simulink library "pixhawk_slib_adv"  (R2017b)
settings: Solver=ode45  StartTime=0.0  StopTime=10.0  RelTol=1e-3
undefined symbols (not defined in the file or in its folder): Earth, earthRadius, ModelInit_AngEuler, ModelInit_PosE, ModelInit_RateB, ModelInit_RPM, ModelInit_VelB, ModelParam_envAltitude, ModelParam_GPSLatLong, ModelParam_motorCr, ModelParam_motorJm, ModelParam_motorT, ModelParam_motorWb, ModelParam_noisePowerIMU, ModelParam_rotorCm, ModelParam_rotorCt, ModelParam_uavCCm, ModelParam_uavCd, ModelParam_uavDearo, ModelParam_uavJ, ModelParam_uavMass, ModelParam_uavR, ModelParam_uavType, Receive, Send, WGS84
libraries: etargetslib x11, dspnetwork x9, simulink x8, sharedtransform x5, aerolibtransform2 x4, aerolibutil x4, pixhawk_slib_adv x3, aerolibfltsims x3, shared6dof x1, aerolibobsolete x1, aerolibasang x1, aerolibatmos2 x1
(part 1 of 3)
settings Model: Creator=skuznick  LastModifiedBy=uavcs
settings DataIOCC: LimitDataPoints=on  SaveFormat=Array
settings OptimizationCC: BlockReduction=off  BooleanDataType=off  LifeSpan=inf
settings DebuggingCC: SaveWithParameterizedLinksMsg=none  UnderspecifiedInitializationDetection=Classic  MergeDetectMultiDrivingBlocksExec=none  SignalResolutionControl=TryResolveAllWithWarning  AllowSymbolicDim=off  SFUnexpectedBacktrackingDiag=warning  SFNoUnconditionalDefaultTransitionDiag=warning  SFExecutionAtInitializationDiag=none
settings HardwareCC: ProdBitPerPointer=32  ProdBitPerSizeT=32  ProdBitPerPtrDiffT=32  ProdLargestAtomicFloat=None  ProdIntDivRoundTo=Undefined  ProdEndianess=Unspecified  ProdWordSize=32  ProdHWDeviceType=32-bit Generic  TargetUnknown=on
settings ModelReferenceCC: PropagateSignalLabelsOutOfModel=off
settings CodeAppCC: StateflowObjectComments=on
settings GRTTargetCC: TargetLangStandard=C89/C90 (ANSI)
settings ConfigComp: CovMetricSettings=dw  CovSaveCumulativeToWorkspaceVar=on  CovSaveSingleToWorkspaceVar=on  CovExternalEMLEnable=off  CovSFcnEnable=off

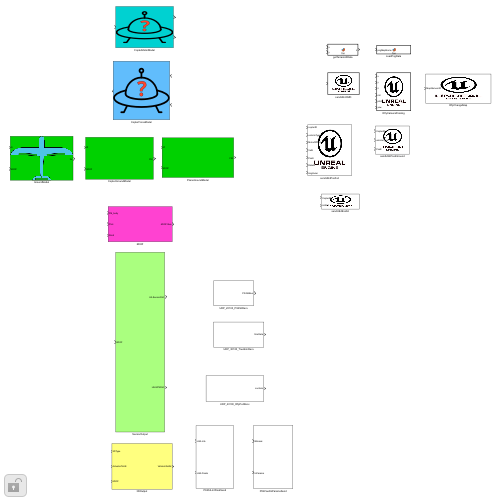
[thumbnail: Simulink's stored preview of the top-level diagram]
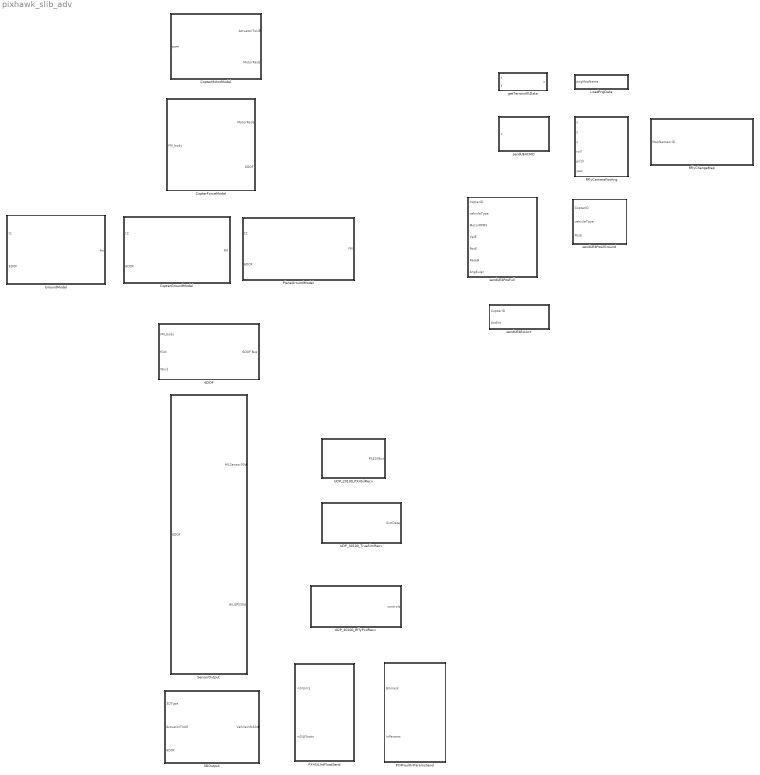
== system pixhawk_slib_adv ==
  3DOutput : Subsystem  mask(3DOutput API){}
      mask help:
      | 该模块输入为：
      | 1）UAVType：三维显示ID，来自***_init.m中的ModelParam_uavType，由三维模型文件中的XML文件决定，例如：常规四旋翼的UAVType为3，小型固定翼的UAVType为100。
      | 2）ActuatorToUE：来自电机模型，决定了在三维引擎中无人载具系统电机/舵机的转动情况。
      | 3）6DOF：来自6DOF模型的6DOF Bus输入，接收无人载具系统的位置、速度、姿态和加速度等信息。
      | 输出为VehileInfo60d：在三维显示模块中，会通过该接口将数据发送至三维引擎，实现可视化处理。
      mask Help: eval('sharedhelp(''3doutput'')');
      mask DialogControl Control3 Prompt: 模块详解
      mask DialogControl Control3 Callback: !start ../html/md_ctrl_2md_23DOutput.html
      mask DialogControl Control2 Prompt: (Add text here)
  6DOF : Subsystem  mask(6DOF API){Init_PosE=ModelInit_PosE, Init_VelB=ModelInit_VelB, Init_AngEuler=ModelInit_AngEuler, Init_RateB=ModelInit_RateB, Param_uavMass=ModelParam_uavMass, Param_uavJ=ModelParam_uavJ, Param_GPSLatLong=ModelParam_GPSLatLong, Param_envAltitude=ModelParam_envAltitude}
      mask prompts: Init_PosE "Initial position NED:"; Init_VelB "Initial velocity FRD:"; Init_AngEuler "Initial Euler Ang:"; Init_RateB "Initial Ang Rate:"; Param_uavMass "Vehilce Mass:"; Param_uavJ "Vehicle Inertial Matrix:"; Param_GPSLatLong "Gps Initial Lat and Lon:"; Param_envAltitude "Gps Init Alt:"
      mask help:
      | 该模块中包括了环境模型和基于四元数的刚体六自由度模型。环境模型对重力和大气压强对无人系统飞行产生的影响进行了模拟；刚体六自由度模型用于描述无人载具运动时的姿态和位置变化
      | 以旋翼无人机为例，六自由度模块基于刚体动力学原理，将无人机视为一个刚体，并考虑了无人机在三个坐标轴上的旋转运动（俯仰、横滚和偏航）以及机体与地球坐标系上的平移运动（前后、左右和上下）。
      | 该模块通过对这些自由度进行数学建模，可以推导出无人机在空中运动时的动力学方程，从而可以进行控制系统设计、路径规划和飞行模拟等应用。此外，还可以根据实际需求对模型进行扩展，考虑更多的因素，如飞行器的非线性特性、气动力和惯性矩等。
      | 该模型的输入为机体所受的力和力矩，输出为机体坐标系下的速度与加速度，地球坐标系下的速度，位置，欧拉角，方向余弦矩阵（旋转矩阵），角速度与角加速度。
      mask Help: eval('sharedhelp(''6dof'')');
      mask DialogControl Control2 Prompt: 模块详解
      mask DialogControl Control2 Callback: !start ../html/md_ctrl_2md_26DOF.html
  CopterForceModel : Subsystem  mask(CopterForceModel){AirframeChoice=default, Param_uavType=ModelParam_uavType, Param_uavR=ModelParam_uavR, Param_motorJm=ModelParam_motorJm, Param_rotorCm=ModelParam_rotorCm, Param_rotorCt=ModelParam_rotorCt, Param_uavCd=ModelParam_uavCd, Param_uavCCm=ModelParam_uavCCm, Param_uavDearo=ModelParam_uavDearo}
      mask prompts: Param_uavType "Uav type id:"; Param_uavR "Airframe size:"; Param_motorJm "Propeller Jm:"; Param_rotorCm "Propeller Cm:"; Param_rotorCt "Propeller Ct:"; Param_uavCd "Uav Cd:"; Param_uavCCm "Uav Cm:"; Param_uavDearo "Uav d_aero:"
      mask help: 力和力矩子系统主要用于综合执行器状态、飞行环境状态和机体运动状态，来计算出机身子系统受到的合力和力矩。为了方便六自由度机体运动模型的使用，合力和力矩通常需要统一映射（坐标转换）到机体坐标系中。
      mask init:
      | choice = get_param(gcb, 'AirframeChoice');
      | switch choice
      |     case 'default'
      |         set_param(gcb, 'Param_uavType', 'ModelParam_uavType');
      |         set_param(gcb, 'Param_uavR', 'ModelParam_uavR');
      |         set_param(gcb, 'Param_motorJm', 'ModelParam_motorJm');
      |         set_param(gcb, 'Param_rotorCm', 'ModelParam_rotorCm');
      |         set_param(gcb, 'Param_rotorCt', 'ModelParam_rotorCt');
      |         set_param(gcb, 'Param_uavCd', 'ModelParam_uavCd');
      |         set_param(gcb, 'Param_uavDearo', 'ModelParam_uavDearo');
      |         set_param(gcb, 'Param_uavCCm', 'ModelParam_uavCCm');
      |     case 'Tricopter Y+'
      |         Param_uavType=int16(1)
      |         Param_uavR=0.225
      |         Param_motorJm=2.13e-4
      |         Param_rotorCm=1.789e-7
      |         Param_rotorCt=1.051e-5
      |         Param_uavCd=0.227
      |         Param_uavDearo=0.12
      |         Param_uavCCm=[0.0035; 0.0039; 0.0034]
      |         set_param(gcb, 'Param_uavCCm', mat2str(Param_uavCCm,'class'));
      |         set_param(gcb, 'Param_uavType', num2str(Param_uavType));
      |         set_param(gcb, 'Param_uavR', num2str(Param_uavR));
      |         set_param(gcb, 'Param_motorJm', num2str(Param_motorJm));
      |         set_param(gcb, 'Param_rotorCm', num2str(Param_rotorCm));
      |         set_param(gcb, 'Param_rotorCt', num2str(Param_rotorCt));
      |         set_param(gcb, 'Param_uavCd', num2str(Param_uavCd));
      |         set_param(gcb, 'Param_uavDearo', num2str(Param_uavDearo));
      |     case 'Tricopter Y-'
      |         Param_uavType=int16(2)
      |         Param_uavR=0.225
      |         Param_motorJm=2.13e-4
      |         Param_rotorCm=1.789e-7
      |         Param_rotorCt=1.051e-5
      |         Param_uavCd=0.227
      |         Param_uavDearo=0.12
      |         Param_uavCCm=[0.0035; 0.0039; 0.0034]
      |         set_param(gcb, 'Param_uavCCm', mat2str(Param_uavCCm,'class'));
      |         set_param(gcb, 'Param_uavType', num2str(Param_uavType));
      |         set_param(gcb, 'Param_uavR', num2str(Param_uavR));
      |         set_param(gcb, 'Param_motorJm', num2str(Param_motorJm));
      |         set_param(gcb, 'Param_rotorCm', num2str(Param_rotorCm));
      |         set_param(gcb, 'Param_rotorCt', num2str(Param_rotorCt));
      |         set_param(gcb, 'Param_uavCd', num2str(Param_uavCd));
      |         set_param(gcb, 'Param_uavDearo', num2str(Param_uavDearo));
      |     case 'Quadrotor X'
      |         Param_uavType=int16(3)
      |         Param_uavR=0.225
      |         Param_motorJm=0.0001287
      |         Param_rotorCm=2.783e-07
      |         Param_rotorCt=1.681e-05
      |         Param_uavCd=0.055
      |         Param_uavDearo=0.12
      |         Param_uavCCm=[0.0035; 0.0039; 0.0034]
      |         set_param(gcb, 'Param_uavCCm', mat2str(Param_uavCCm,'class'));
      |         set_param(gcb, 'Param_uavType', num2str(Param_uavType));
      |         set_param(gcb, 'Param_uavR', num2str(Param_uavR));
      |         set_param(gcb, 'Param_motorJm', num2str(Param_motorJm));
      |         set_param(gcb, 'Param_rotorCm', num2str(Param_rotorCm));
      |         set_param(gcb, 'Param_rotorCt', num2str(Param_rotorCt));
      |         set_param(gcb, 'Param_uavCd', num2str(Param_uavCd));
      |         set_param(gcb, 'Param_uavDearo', num2str(Param_uavDearo));
      |     case 'Quadrotor +'
      |         Param_uavType=int16(4)
      |         Param_uavR=0.225
      |         Param_motorJm=0.0001287
      |         Param_rotorCm=2.783e-07
      |         Param_rotorCt=1.681e-05
      |         Param_uavCd=0.055
      |         Param_uavDearo=0.12
      |         Param_uavCCm=[0.0035; 0.0039; 0.0034]
      |         set_param(gcb, 'Param_uavCCm', mat2str(Param_uavCCm,'class'));
      |         set_param(gcb, 'Param_uavType', num2str(Param_uavType));
      |         set_param(gcb, 'Param_uavR', num2str(Param_uavR));
      |         set_param(gcb, 'Param_motorJm', num2str(Param_motorJm));
      |         set_param(gcb, 'Param_rotorCm', num2str(Param_rotorCm));
      |         set_param(gcb, 'Param_rotorCt', num2str(Param_rotorCt));
      |         set_param(gcb, 'Param_uavCd', num2str(Param_uavCd));
      |         set_param(gcb, 'Param_uavDearo', num2str(Param_uavDearo));
      |     case 'Hexarotor x'
      |         Param_uavType=int16(5)
      |         Param_uavR=0.275
      |         Param_motorJm=2.13e-4
      |         Param_rotorCm=1.789e-7 
      |         Param_rotorCt=1.051e-5 
      |         Param_uavCd=0.339
      |         Param_uavDearo=0.12
      |         Param_uavCCm=[0.0035; 0.0039; 0.0034]
      |         set_param(gcb, 'Param_uavCCm', mat2str(Param_uavCCm,'class'));
      |         set_param(gcb, 'Param_uavType', num2str(Param_uavType));
      |         set_param(gcb, 'Param_uavR', num2str(Param_uavR));
      |         set_param(gcb, 'Param_motorJm', num2str(Param_motorJm));
      |         set_param(gcb, 'Param_rotorCm', num2str(Param_rotorCm));
      |         set_param(gcb, 'Param_rotorCt', num2str(Param_rotorCt));
      |         set_param(gcb, 'Param_uavCd', num2str(Param_uavCd));
      |         set_param(gcb, 'Param_uavDearo', num2str(Param_uavDearo));
      |     case 'Hexarotor +'
      |         Param_uavType=int16(6)
      |         Param_uavR=0.275
      |         Param_motorJm=2.13e-4
      |         Param_rotorCm=1.789e-7 
      |         Param_rotorCt=1.051e-5 
      |         Param_uavCd=0.339
      |         Param_uavDearo=0.12
      |         Param_uavCCm=[0.0035; 0.0039; 0.0034]
      |         set_param(gcb, 'Param_uavCCm', mat2str(Param_uavCCm,'class'));
      |         set_param(gcb, 'Param_uavType', num2str(Param_uavType));
      |         set_param(gcb, 'Param_uavR', num2str(Param_uavR));
      |         set_param(gcb, 'Param_motorJm', num2str(Param_motorJm));
      |         set_param(gcb, 'Param_rotorCm', num2str(Param_rotorCm));
      |         set_param(gcb, 'Param_rotorCt', num2str(Param_rotorCt));
      |         set_param(gcb, 'Param_uavCd', num2str(Param_uavCd));
      |         set_param(gcb, 'Param_uavDearo', num2str(Param_uavDearo));
      |     case 'Hexarotor Coaxial'
      |         Param_uavType=int16(7)
      |         Param_uavR=0.225
      |         Param_motorJm=2.13e-4 
      |         Param_rotorCm=1.789e-7
      |         Param_rotorCt=1.051e-5
      |         Param_uavCd=0.228 
      |         Param_uavDearo=0.12
      |         Param_uavCCm=[0.0035; 0.0039; 0.0034]
      |         set_param(gcb, 'Param_uavCCm', mat2str(Param_uavCCm,'class'));
      |         set_param(gcb, 'Param_uavType', num2str(Param_uavType));
      |         set_param(gcb, 'Param_uavR', num2str(Param_uavR));
      |         set_param(gcb, 'Param_motorJm', num2str(Param_motorJm));
      |         set_param(gcb, 'Param_rotorCm', num2str(Param_rotorCm));
      |         set_param(gcb, 'Param_rotorCt', num2str(Param_rotorCt));
      |         set_param(gcb, 'Param_uavCd', num2str(Param_uavCd));
      |         set_param(gcb, 'Param_uavDearo', num2str(Param_uavDearo));
      |     case 'Octorotor x'
      |         Param_uavType=int16(8)
      |         Param_uavR=0.325
      |         Param_motorJm= 8.00e-5 
      |         Param_rotorCm= 1.417e-7
      |         Param_rotorCt=8.380e-6
      |         Param_uavCd=0.472
      |         Param_uavDearo=0.12
      |         Param_uavCCm=[0.0035; 0.0039; 0.0034]
      |         set_param(gcb, 'Param_uavCCm', mat2str(Param_uavCCm,'class'));
      |         set_param(gcb, 'Param_uavType', num2str(Param_uavType));
      |         set_param(gcb, 'Param_uavR', num2str(Param_uavR));
      |         set_param(gcb, 'Param_motorJm', num2str(Param_motorJm));
      |         set_param(gcb, 'Param_rotorCm', num2str(Param_rotorCm));
      |         set_param(gcb, 'Param_rotorCt', num2str(Param_rotorCt));
      |         set_param(gcb, 'Param_uavCd', num2str(Param_uavCd));
      |         set_param(gcb, 'Param_uavDearo', num2str(Param_uavDearo));
      |     case 'Octorotor +'
      |         Param_uavType=int16(9)
      |         Param_uavR=0.325
      |         Param_motorJm= 8.00e-5 
      |         Param_rotorCm= 1.417e-7
      |         Param_rotorCt=8.380e-6
      |         Param_uavCd=0.472
      |         Param_uavDearo=0.12
      |         Param_uavCCm=[0.0035; 0.0039; 0.0034]
      |         set_param(gcb, 'Param_uavCCm', mat2str(Param_uavCCm,'class'));
      |         set_param(gcb, 'Param_uavType', num2str(Param_uavType));
      |         set_param(gcb, 'Param_uavR', num2str(Param_uavR));
      |         set_param(gcb, 'Param_motorJm', num2str(Param_motorJm));
      |         set_param(gcb, 'Param_rotorCm', num2str(Param_rotorCm));
      |         set_param(gcb, 'Param_rotorCt', num2str(Param_rotorCt));
      |         set_param(gcb, 'Param_uavCd', num2str(Param_uavCd));
      |         set_param(gcb, 'Param_uavDearo', num2str(Param_uavDearo));
      |     case 'Octorotor Coaxial'
      |         Param_uavType=int16(10)
      |         Param_uavR=0.275
      |         Param_motorJm=2.13e-4 
      |         Param_rotorCm=1.789e-7 
      |         Param_rotorCt=1.051e-5 
      |         Param_uavCd=0.338
      |         Param_uavDearo=0.12
      |         Param_uavCCm=[0.0035; 0.0039; 0.0034]
      |         set_param(gcb, 'Param_uavCCm', mat2str(Param_uavCCm,'class'));
      |         set_param(gcb, 'Param_uavType', num2str(Param_uavType));
      |         set_param(gcb, 'Param_uavR', num2str(Param_uavR));
      |         set_param(gcb, 'Param_motorJm', num2str(Param_motorJm));
      |         set_param(gcb, 'Param_rotorCm', num2str(Param_rotorCm));
      |         set_param(gcb, 'Param_rotorCt', num2str(Param_rotorCt));
      |         set_param(gcb, 'Param_uavCd', num2str(Param_uavCd));
      |         set_param(gcb, 'Param_uavDearo', num2str(Param_uavDearo)); 
      |     otherwise
      |         error('Unknown AirframeChoice');
      | end
      | 
      | % 更新Param_uavType参数值
      | 
      | % 显示更新后的值在mask界面上（假设你有一个显示区域来展示此值）
      | disp(['Updated Param_uavType: ', num2str(Param_uavType)]);
      mask Help: eval('sharedhelp(''copterforce'')');
      mask TypeOptions AirframeChoice: default | Tricopter Y+ | Tricopter Y- | Quadrotor X | Quadrotor + | Hexarotor x | Hexarotor + | Hexarotor Coaxial | Octorotor x | Octorotor + | Octorotor Coaxial
      mask Callback AirframeChoice:
      | choice = get_param(gcb, 'AirframeChoice');
      | switch choice
      |     case 'default'
      |         set_param(gcb, 'Param_uavType', 'ModelParam_uavType');
      |         set_param(gcb, 'Param_uavR', 'ModelParam_uavR');
      |         set_param(gcb, 'Param_motorJm', 'ModelParam_motorJm');
      |         set_param(gcb, 'Param_rotorCm', 'ModelParam_rotorCm');
      |         set_param(gcb, 'Param_rotorCt', 'ModelParam_rotorCt');
      |         set_param(gcb, 'Param_uavCd', 'ModelParam_uavCd');
      |         set_param(gcb, 'Param_uavDearo', 'ModelParam_uavDearo');
      |         set_param(gcb, 'Param_uavCCm', 'ModelParam_uavCCm');
      |     case 'Tricopter Y+'
      |         Param_uavType=1
      |         Param_uavR=0.225
      |         Param_motorJm=2.13e-4
      |         Param_rotorCm=1.789e-7
      |         Param_rotorCt=1.051e-5
      |         Param_uavCd=0.227
      |         Param_uavDearo=0.12
      |         Param_uavCCm=[0.0035; 0.0039; 0.0034]
      |         set_param(gcb, 'Param_uavCCm', mat2str(Param_uavCCm,'class'));
      |         set_param(gcb, 'Param_uavType', num2str(Param_uavType));
      |         set_param(gcb, 'Param_uavR', num2str(Param_uavR));
      |         set_param(gcb, 'Param_motorJm', num2str(Param_motorJm));
      |         set_param(gcb, 'Param_rotorCm', num2str(Param_rotorCm));
      |         set_param(gcb, 'Param_rotorCt', num2str(Param_rotorCt));
      |         set_param(gcb, 'Param_uavCd', num2str(Param_uavCd));
      |         set_param(gcb, 'Param_uavDearo', num2str(Param_uavDearo));
      |     case 'Tricopter Y-'
      |         Param_uavType=2
      |         Param_uavR=0.225
      |         Param_motorJm=2.13e-4
      |         Param_rotorCm=1.789e-7
      |         Param_rotorCt=1.051e-5
      |         Param_uavCd=0.227
      |         Param_uavDearo=0.12
      |         Param_uavCCm=[0.0035; 0.0039; 0.0034]
      |         set_param(gcb, 'Param_uavCCm', mat2str(Param_uavCCm,'class'));
      |         set_param(gcb, 'Param_uavType', num2str(Param_uavType));
      |         set_param(gcb, 'Param_uavR', num2str(Param_uavR));
      |         set_param(gcb, 'Param_motorJm', num2str(Param_motorJm));
      |         set_param(gcb, 'Param_rotorCm', num2str(Param_rotorCm));
      |         set_param(gcb, 'Param_rotorCt', num2str(Param_rotorCt));
      |         set_param(gcb, 'Param_uavCd', num2str(Param_uavCd));
      |         set_param(gcb, 'Param_uavDearo', num2str(Param_uavDearo));
      |     case 'Quadrotor X'
      |         Param_uavType=3
      |         Param_uavR=0.225
      |         Param_motorJm=0.0001287
      |         Param_rotorCm=2.783e-07
      |         Param_rotorCt=1.681e-05
      |         Param_uavCd=0.055
      |         Param_uavDearo=0.12
      |         Param_uavCCm=[0.0035; 0.0039; 0.0034]
      |         set_param(gcb, 'Param_uavCCm', mat2str(Param_uavCCm,'class'));
      |         set_param(gcb, 'Param_uavType', num2str(Param_uavType));
      |         set_param(gcb, 'Param_uavR', num2str(Param_uavR));
      |         set_param(gcb, 'Param_motorJm', num2str(Param_motorJm));
      |         set_param(gcb, 'Param_rotorCm', num2str(Param_rotorCm));
      |         set_param(gcb, 'Param_rotorCt', num2str(Param_rotorCt));
      |         set_param(gcb, 'Param_uavCd', num2str(Param_uavCd));
      |         set_param(gcb, 'Param_uavDearo', num2str(Param_uavDearo));
      |     case 'Quadrotor +'
      |         Param_uavType=4
      |         Param_uavR=0.225
      |         Param_motorJm=0.0001287
      |         Param_rotorCm=2.783e-07
      |         Param_rotorCt=1.681e-05
      |         Param_uavCd=0.055
      |         Param_uavDearo=0.12
      |         Param_uavCCm=[0.0035; 0.0039; 0.0034]
      |         set_param(gcb, 'Param_uavCCm', mat2str(Param_uavCCm,'class'));
      |         set_param(gcb, 'Param_uavType', num2str(Param_uavType));
      |         set_param(gcb, 'Param_uavR', num2str(Param_uavR));
      |         set_param(gcb, 'Param_motorJm', num2str(Param_motorJm));
      |         set_param(gcb, 'Param_rotorCm', num2str(Param_rotorCm));
      |         set_param(gcb, 'Param_rotorCt', num2str(Param_rotorCt));
      |         set_param(gcb, 'Param_uavCd', num2str(Param_uavCd));
      |         set_param(gcb, 'Param_uavDearo', num2str(Param_uavDearo));
      |     case 'Hexarotor x'
      |         Param_uavType=5
      |         Param_uavR=0.275
      |         Param_motorJm=2.13e-4
      |         Param_rotorCm=1.789e-7
      |         Param_rotorCt=1.051e-5
      |         Param_uavCd=0.339
      |         Param_uavDearo=0.12
      |         Param_uavCCm=[0.0035; 0.0039; 0.0034]
      |         set_param(gcb, 'Param_uavCCm', mat2str(Param_uavCCm,'class'));
      |         set_param(gcb, 'Param_uavType', num2str(Param_uavType));
      |         set_param(gcb, 'Param_uavR', num2str(Param_uavR));
      |         set_param(gcb, 'Param_motorJm', num2str(Param_motorJm));
      |         set_param(gcb, 'Param_rotorCm', num2str(Param_rotorCm));
      |         set_param(gcb, 'Param_rotorCt', num2str(Param_rotorCt));
      |         set_param(gcb, 'Param_uavCd', num2str(Param_uavCd));
      |         set_param(gcb, 'Param_uavDearo', num2str(Param_uavDearo));
      |     case 'Hexarotor +'
      |         Param_uavType=6
      |         Param_uavR=0.275
      |         Param_motorJm=2.13e-4
      |         Param_rotorCm=1.789e-7
      |         Param_rotorCt=1.051e-5
      |         Param_uavCd=0.339
      |         Param_uavDearo=0.12
      |         Param_uavCCm=[0.0035; 0.0039; 0.0034]
      |         set_param(gcb, 'Param_uavCCm', mat2str(Param_uavCCm,'class'));
      |         set_param(gcb, 'Param_uavType', num2str(Param_uavType));
      |         set_param(gcb, 'Param_uavR', num2str(Param_uavR));
      |         set_param(gcb, 'Param_motorJm', num2str(Param_motorJm));
      |         set_param(gcb, 'Param_rotorCm', num2str(Param_rotorCm));
      |         set_param(gcb, 'Param_rotorCt', num2str(Param_rotorCt));
      |         set_param(gcb, 'Param_uavCd', num2str(Param_uavCd));
      |         set_param(gcb, 'Param_uavDearo', num2str(Param_uavDearo));
      |     case 'Hexarotor Coaxial'
      |         Param_uavType=7
      |         Param_uavR=0.225
      |         Param_motorJm=2.13e-4
      |         Param_rotorCm=1.789e-7
      |         Param_rotorCt=1.051e-5
      |         Param_uavCd=0.228
      |         Param_uavDearo=0.12
      |         Param_uavCCm=[0.0035; 0.0039; 0.0034]
      |         set_param(gcb, 'Param_uavCCm', mat2str(Param_uavCCm,'class'));
      |         set_param(gcb, 'Param_uavType', num2str(Param_uavType));
      |         set_param(gcb, 'Param_uavR', num2str(Param_uavR));
      |         set_param(gcb, 'Param_motorJm', num2str(Param_motorJm));
      |         set_param(gcb, 'Param_rotorCm', num2str(Param_rotorCm));
      |         set_param(gcb, 'Param_rotorCt', num2str(Param_rotorCt));
      |         set_param(gcb, 'Param_uavCd', num2str(Param_uavCd));
      |         set_param(gcb, 'Param_uavDearo', num2str(Param_uavDearo));
      |     case 'Octorotor x'
      |         Param_uavType=8
      |         Param_uavR=0.325
      |         Param_motorJm= 8.00e-5
      |         Param_rotorCm= 1.417e-7
      |         Param_rotorCt=8.380e-6
      |         Param_uavCd=0.472
      |         Param_uavDearo=0.12
      |         Param_uavCCm=[0.0035; 0.0039; 0.0034]
      |         set_param(gcb, 'Param_uavCCm', mat2str(Param_uavCCm,'class'));
      |         set_param(gcb, 'Param_uavType', num2str(Param_uavType));
      |         set_param(gcb, 'Param_uavR', num2str(Param_uavR));
      |         set_param(gcb, 'Param_motorJm', num2str(Param_motorJm));
      |         set_param(gcb, 'Param_rotorCm', num2str(Param_rotorCm));
      |         set_param(gcb, 'Param_rotorCt', num2str(Param_rotorCt));
      |         set_param(gcb, 'Param_uavCd', num2str(Param_uavCd));
      |         set_param(gcb, 'Param_uavDearo', num2str(Param_uavDearo));
      |     case 'Octorotor +'
      |         Param_uavType=9
      |         Param_uavR=0.325
      |         Param_motorJm= 8.00e-5
      |         Param_rotorCm= 1.417e-7
      |         Param_rotorCt=8.380e-6
      |         Param_uavCd=0.472
      |         Param_uavDearo=0.12
      |         Param_uavCCm=[0.0035; 0.0039; 0.0034]
      |         set_param(gcb, 'Param_uavCCm', mat2str(Param_uavCCm,'class'));
      |         set_param(gcb, 'Param_uavType', num2str(Param_uavType));
      |         set_param(gcb, 'Param_uavR', num2str(Param_uavR));
      |         set_param(gcb, 'Param_motorJm', num2str(Param_motorJm));
      |         set_param(gcb, 'Param_rotorCm', num2str(Param_rotorCm));
      |         set_param(gcb, 'Param_rotorCt', num2str(Param_rotorCt));
      |         set_param(gcb, 'Param_uavCd', num2str(Param_uavCd));
      |         set_param(gcb, 'Param_uavDearo', num2str(Param_uavDearo));
      |     case 'Octorotor Coaxial'
      |         Param_uavType=10
      |         Param_uavR=0.275
      |         Param_motorJm=2.13e-4
      |         Param_rotorCm=1.789e-7
      |         Param_rotorCt=1.051e-5
      |         Param_uavCd=0.338
      |         Param_uavDearo=0.12
      |         Param_uavCCm=[0.0035; 0.0039; 0.0034]
      |         set_param(gcb, 'Param_uavCCm', mat2str(Param_uavCCm,'class'));
      |         set_param(gcb, 'Param_uavType', num2str(Param_uavType));
      |         set_param(gcb, 'Param_uavR', num2str(Param_uavR));
      |         set_param(gcb, 'Param_motorJm', num2str(Param_motorJm));
      |         set_param(gcb, 'Param_rotorCm', num2str(Param_rotorCm));
      |         set_param(gcb, 'Param_rotorCt', num2str(Param_rotorCt));
      |         set_param(gcb, 'Param_uavCd', num2str(Param_uavCd));
      |         set_param(gcb, 'Param_uavDearo', num2str(Param_uavDearo));
      |     otherwise
      |         error('Unknown AirframeChoice');
      | end
      mask DialogControl Control2 Prompt: 模块详解
      mask DialogControl Control2 Callback: !start ../html/md_ctrl_2md_2CopterForceModel.html
      mask Display:
      | choice = get_param(gcb, 'AirframeChoice');
      | if strcmp(choice, 'Tricopter Y+')
      |     image('YPlus.svg'); % 图标1
      | elseif strcmp(choice, 'Tricopter Y-')
      |     image('Ymin.svg'); % 图标2
      | elseif strcmp(choice, 'Quadrotor X')
      |     image('QuadRotorX.svg'); % 图标3
      | elseif strcmp(choice, 'Quadrotor +')
      |     image('QuadRotorPlus.svg'); % 图标4
      | elseif strcmp(choice, 'Hexarotor x')
      |     image('HexaRotorX.svg'); % 图标5
      | elseif strcmp(choice, 'Hexarotor +')
      |     image('HexaRotorPlus.svg'); % 图标6
      | elseif strcmp(choice, 'Hexarotor Coaxial')
      |     image('Y6B.svg'); % 图标7
      | elseif strcmp(choice, 'Octorotor x')
      |     image('OctoRotorX.svg'); % 图标8
      | elseif strcmp(choice, 'Octorotor +')
      |     image('OctoRotorPlus.svg'); % 图标9
      | elseif strcmp(choice, 'Octorotor Coaxial')
      |     image('OctoRotorXCoaxial.svg'); % 图标10
      | else
      |     image('default.svg'); % 默认图标
      | end
  CopterGroundModel : Subsystem  mask(CopterGroundModel){}
      mask help: 旋翼类的地面挤压和摩擦模型
      mask Help: eval('sharedhelp(''groundmodel'')');
      mask DialogControl Control3 Prompt: 模块详解
      mask DialogControl Control3 Callback: !start ../html/md_ctrl_2md_2GroundModel.html
      mask DialogControl Control2 Prompt: (Add text here)
  CopterMotorModel : Subsystem  mask(CopterMotorModel){AirframeChoice=default, Param_motorWb=ModelParam_motorWb, Param_motorCr=ModelParam_motorCr, Param_motorT=ModelParam_motorT, ModelParam_motorMinThr=0.05}
      mask prompts: Param_motorWb "Motor Wb:"; Param_motorCr "Motor Cr:"; Param_motorT "Motor T:"; ModelParam_motorMinThr "Motor min thr:"
      mask help: 多旋翼电机通常由电机本体、转子、定子和控制器组成。转子上的螺旋桨通过电机转动产生升力和推力，而控制器则负责调节电机的速度和方向。从而实现无人机的稳定悬停、前进、后退、转向等动作。在该模块中输入为PWM值，经过各电机的非线性动力学模型后得到各电机转速，该模块的输出分别为输入给力和力矩模型的电机转速（弧度每秒）；输入给UE的电机转速（转每分），由于UE中多旋翼的三维模型输入单位为转每分，所以在传输给UE的转速上做了单位转换。
      mask init:
      | choice = get_param(gcb, 'AirframeChoice');
      | switch choice
      |     case 'default'
      |         set_param(gcb, 'Param_motorWb', 'ModelParam_motorWb');
      |         set_param(gcb, 'Param_motorCr', 'ModelParam_motorCr');
      |         set_param(gcb, 'Param_motorT', 'ModelParam_motorT');
      |     case 'Tricopter Y+'
      |         Param_motorWb=147.17
      |         Param_motorCr=757.47 
      |         Param_motorT=  0.0899
      |         set_param(gcb, 'Param_motorWb', num2str(Param_motorWb));
      |         set_param(gcb, 'Param_motorCr', num2str(Param_motorCr));
      |         set_param(gcb, 'Param_motorT', num2str(Param_motorT));
      |     case 'Tricopter Y-'
      |         Param_motorWb=147.17
      |         Param_motorCr=757.47 
      |         Param_motorT=  0.0899 
      |         set_param(gcb, 'Param_motorWb', num2str(Param_motorWb));
      |         set_param(gcb, 'Param_motorCr', num2str(Param_motorCr));
      |         set_param(gcb, 'Param_motorT', num2str(Param_motorT));
      |     case 'Quadrotor X'
      |         Param_motorWb=22.83
      |         Param_motorCr=842.1
      |         Param_motorT=0.0214
      |         set_param(gcb, 'Param_motorWb', num2str(Param_motorWb));
      |         set_param(gcb, 'Param_motorCr', num2str(Param_motorCr));
      |         set_param(gcb, 'Param_motorT', num2str(Param_motorT));
      |     case 'Quadrotor +'
      |         Param_motorWb=22.83
      |         Param_motorCr=842.1
      |         Param_motorT=0.0214
      |         set_param(gcb, 'Param_motorWb', num2str(Param_motorWb));
      |         set_param(gcb, 'Param_motorCr', num2str(Param_motorCr));
      |         set_param(gcb, 'Param_motorT', num2str(Param_motorT));
      |     case 'Hexarotor x'
      |         Param_motorWb=131.17
      |         Param_motorCr=661.53
      |         Param_motorT=0.0892
      |         set_param(gcb, 'Param_motorWb', num2str(Param_motorWb));
      |         set_param(gcb, 'Param_motorCr', num2str(Param_motorCr));
      |         set_param(gcb, 'Param_motorT', num2str(Param_motorT));
      |     case 'Hexarotor +'
      |         Param_motorWb=131.17
      |         Param_motorCr=661.53
      |         Param_motorT=0.0892
      |         set_param(gcb, 'Param_motorWb', num2str(Param_motorWb));
      |         set_param(gcb, 'Param_motorCr', num2str(Param_motorCr));
      |         set_param(gcb, 'Param_motorT', num2str(Param_motorT));
      |     case 'Hexarotor Coaxial'
      |         Param_motorWb=137.45  
      |         Param_motorCr=670.36 
      |         Param_motorT= 0.0884
      |         set_param(gcb, 'Param_motorWb', num2str(Param_motorWb));
      |         set_param(gcb, 'Param_motorCr', num2str(Param_motorCr));
      |         set_param(gcb, 'Param_motorT', num2str(Param_motorT));
      |     case 'Octorotor x'
      |         Param_motorWb=108.72
      |         Param_motorCr=718.43
      |         Param_motorT=0.034
      |         set_param(gcb, 'Param_motorWb', num2str(Param_motorWb));
      |         set_param(gcb, 'Param_motorCr', num2str(Param_motorCr));
      |         set_param(gcb, 'Param_motorT', num2str(Param_motorT));
      |     case 'Octorotor +'
      |         Param_motorWb=108.72
      |         Param_motorCr=718.43
      |         Param_motorT=0.034
      |         set_param(gcb, 'Param_motorWb', num2str(Param_motorWb));
      |         set_param(gcb, 'Param_motorCr', num2str(Param_motorCr));
      |         set_param(gcb, 'Param_motorT', num2str(Param_motorT));
      |     case 'Octorotor Coaxial'
      |         Param_motorWb=129.39 
      |         Param_motorCr=658.62 
      |         Param_motorT=0.0894 
      |         set_param(gcb, 'Param_motorWb', num2str(Param_motorWb));
      |         set_param(gcb, 'Param_motorCr', num2str(Param_motorCr));
      |         set_param(gcb, 'Param_motorT', num2str(Param_motorT));
      |     otherwise
      |         error('Unknown AirframeChoice');
      | end
      mask Help: eval('sharedhelp(''coptermotor'')');
      mask TypeOptions AirframeChoice: default | Tricopter Y+ | Tricopter Y- | Quadrotor X | Quadrotor + | Hexarotor x | Hexarotor + | Hexarotor Coaxial | Octorotor x | Octorotor + | Octorotor Coaxial
      mask Callback AirframeChoice:
      | choice = get_param(gcb, 'AirframeChoice');
      | switch choice
      |     case 'default'
      |         set_param(gcb, 'Param_motorWb', 'ModelParam_motorWb');
      |         set_param(gcb, 'Param_motorCr', 'ModelParam_motorCr');
      |         set_param(gcb, 'Param_motorT', 'ModelParam_motorT');
      |     case 'Tricopter Y+'
      |         Param_motorWb=147.17
      |         Param_motorCr=757.47
      |         Param_motorT=  0.0899
      |         set_param(gcb, 'Param_motorWb', num2str(Param_motorWb));
      |         set_param(gcb, 'Param_motorCr', num2str(Param_motorCr));
      |         set_param(gcb, 'Param_motorT', num2str(Param_motorT));
      |     case 'Tricopter Y-'
      |         Param_motorWb=147.17
      |         Param_motorCr=757.47
      |         Param_motorT=  0.0899
      |         set_param(gcb, 'Param_motorWb', num2str(Param_motorWb));
      |         set_param(gcb, 'Param_motorCr', num2str(Param_motorCr));
      |         set_param(gcb, 'Param_motorT', num2str(Param_motorT));
      |     case 'Quadrotor X'
      |         Param_motorWb=22.83
      |         Param_motorCr=842.1
      |         Param_motorT=0.0214
      |         set_param(gcb, 'Param_motorWb', num2str(Param_motorWb));
      |         set_param(gcb, 'Param_motorCr', num2str(Param_motorCr));
      |         set_param(gcb, 'Param_motorT', num2str(Param_motorT));
      |     case 'Quadrotor +'
      |         Param_motorWb=22.83
      |         Param_motorCr=842.1
      |         Param_motorT=0.0214
      |         set_param(gcb, 'Param_motorWb', num2str(Param_motorWb));
      |         set_param(gcb, 'Param_motorCr', num2str(Param_motorCr));
      |         set_param(gcb, 'Param_motorT', num2str(Param_motorT));
      |     case 'Hexarotor x'
      |         Param_motorWb=131.17
      |         Param_motorCr=661.53
      |         Param_motorT=0.0892
      |         set_param(gcb, 'Param_motorWb', num2str(Param_motorWb));
      |         set_param(gcb, 'Param_motorCr', num2str(Param_motorCr));
      |         set_param(gcb, 'Param_motorT', num2str(Param_motorT));
      |     case 'Hexarotor +'
      |         Param_motorWb=131.17
      |         Param_motorCr=661.53
      |         Param_motorT=0.0892
      |         set_param(gcb, 'Param_motorWb', num2str(Param_motorWb));
      |         set_param(gcb, 'Param_motorCr', num2str(Param_motorCr));
      |         set_param(gcb, 'Param_motorT', num2str(Param_motorT));
      |     case 'Hexarotor Coaxial'
      |         Param_motorWb=137.45
      |         Param_motorCr=670.36
      |         Param_motorT= 0.0884
      |         set_param(gcb, 'Param_motorWb', num2str(Param_motorWb));
      |         set_param(gcb, 'Param_motorCr', num2str(Param_motorCr));
      |         set_param(gcb, 'Param_motorT', num2str(Param_motorT));
      |     case 'Octorotor x'
      |         Param_motorWb=108.72
      |         Param_motorCr=718.43
      |         Param_motorT=0.034
      |         set_param(gcb, 'Param_motorWb', num2str(Param_motorWb));
      |         set_param(gcb, 'Param_motorCr', num2str(Param_motorCr));
      |         set_param(gcb, 'Param_motorT', num2str(Param_motorT));
      |     case 'Octorotor +'
      |         Param_motorWb=108.72
      |         Param_motorCr=718.43
      |         Param_motorT=0.034
      |         set_param(gcb, 'Param_motorWb', num2str(Param_motorWb));
      |         set_param(gcb, 'Param_motorCr', num2str(Param_motorCr));
      |         set_param(gcb, 'Param_motorT', num2str(Param_motorT));
      |     case 'Octorotor Coaxial'
      |         Param_motorWb=129.39
      |         Param_motorCr=658.62
      |         Param_motorT=0.0894
      |         set_param(gcb, 'Param_motorWb', num2str(Param_motorWb));
      |         set_param(gcb, 'Param_motorCr', num2str(Param_motorCr));
      |         set_param(gcb, 'Param_motorT', num2str(Param_motorT));
      |     otherwise
      |         error('Unknown AirframeChoice');
      | end
      mask DialogControl Control2 Prompt: 模块详解
      mask DialogControl Control2 Callback: !start ../html/md_ctrl_2md_2CopterMotorModel.html
      mask Display:
      | choice = get_param(gcb, 'AirframeChoice');
      | if strcmp(choice, 'Tricopter Y+')
      |     image('YPlus.svg'); % 图标1
      | elseif strcmp(choice, 'Tricopter Y-')
      |     image('Ymin.svg'); % 图标2
      | elseif strcmp(choice, 'Quadrotor X')
      |     image('QuadRotorX.svg'); % 图标3
      | elseif strcmp(choice, 'Quadrotor +')
      |     image('QuadRotorPlus.svg'); % 图标4
      | elseif strcmp(choice, 'Hexarotor x')
      |     image('HexaRotorX.svg'); % 图标5
      | elseif strcmp(choice, 'Hexarotor +')
      |     image('HexaRotorPlus.svg'); % 图标6
      | elseif strcmp(choice, 'Hexarotor Coaxial')
      |     image('Y6B.svg'); % 图标7
      | elseif strcmp(choice, 'Octorotor x')
      |     image('OctoRotorX.svg'); % 图标8
      | elseif strcmp(choice, 'Octorotor +')
      |     image('OctoRotorPlus.svg'); % 图标9
      | elseif strcmp(choice, 'Octorotor Coaxial')
      |     image('OctoRotorXCoaxial.svg'); % 图标10
      | else
      |     image('default.svg'); % 默认图标
      | end
  GroundModel : Subsystem  mask(GroundModel){SubsystemChoice=plane, ModelChoice=1}
      mask help: 计算地面挤压和摩擦产生的力和力矩
      mask init:
      | % 获取参数值
      | choice = get_param(gcb, 'SubsystemChoice');
      | 
      | % 设置Multiport Switch选择输入
      | if strcmp(choice, 'plane')
      |     set_param(gcb, 'ModelChoice', '1');
      | elseif strcmp(choice, 'QuadRotorX')
      |     set_param(gcb , 'ModelChoice', '2');
      | end
      mask Help: eval('sharedhelp(''groundmodel'')');
      mask TypeOptions SubsystemChoice: plane | QuadRotorX
      mask DialogControl Control2 Prompt: 模块详解
      mask DialogControl Control2 Callback: !start ../html/md_ctrl_2md_2GroundModel.html
      mask Display:
      | choice = get_param(gcb, 'SubsystemChoice');
      |     if strcmp(choice, 'plane')
      |         image('plane.svg'); % 图标1
      |     elseif strcmp(choice, 'QuadRotorX')
      |         image('QuadRotorX.svg'); % 图标2
      |     else
      |         image('defaultIcon.png'); % 默认图标
      |     end
  LoadPngData : MATLAB Function  TreatAsAtomicUnit=on  mask(LoadPngData){}
      mask help: 通过灰度图和校准数据加载地形高程信息到MapHeightData.mat中
  PX4FaultInParamsSend : Subsystem  mask{TargetIP=127.0.0.1, CopterID=1}
      mask prompts: TargetIP "Target IP Address"
      mask Help: eval('sharedhelp(''PX4FaultInParamsSend'')');
  PX4SILIntFloatSend : Subsystem  mask{TargetIP=127.0.0.1, CopterID=1}
      mask prompts: TargetIP "Target IP Address"
      mask Help: eval('sharedhelp(''PX4SILIntFloatSend'')');
  PlaneGroundModel : Subsystem  mask(PlaneGroundModel){}
      mask help: 固定翼类的地面挤压和摩擦模型
      mask Help: eval('sharedhelp(''groundmodel'')');
      mask DialogControl Control3 Prompt: 模块详解
      mask DialogControl Control3 Callback: !start ../html/md_ctrl_2md_2GroundModel.html
      mask DialogControl Control2 Prompt: (Add text here)
  RflyCameraPosAng : MATLAB Function  TreatAsAtomicUnit=on  mask(RflyCameraPosAng){}
      mask help: 调整RflySim3D内视口相机的位置和视角
  RflyChangeMap : Subsystem
      mask Help: eval('sharedhelp(''RflyCameraPosAng'')');
      mask Display: image('UE_Logo.jpg');
  SensorOutput : Subsystem  mask(SensorOutput API){Param_GlobalNoiseGainSwitch=0}
      mask prompts: Param_GlobalNoiseGainSwitch "Noise rate (0-1)"
      mask help:
      | 该模块中包括了传感器模型和GPS模型，其中传感器模型不仅对磁力计、惯性导航进行了建模，同时加入了噪声模拟；GPS模型用于计算GPS数据，在仿真时反馈回PX4控制器。
      | 该模块输入为6DOF Bus结构体，输出为30维的HILSensor向量和30维的HILGPS向量。
      mask Help: eval('sharedhelp(''sensoroutput'')');
      mask DialogControl Control2 Prompt: 模块详解
      mask DialogControl Control2 Callback: !start ../html/md_ctrl_2md_2SensorOutput.html
  UDP_20100_PX4SilRecv : Subsystem  mask{CopterID=1, OrinLatLon=[40.1540302,116.259368300000], OrinAlt=50, SamTime=-1}
      mask prompts: OrinLatLon "GPS Orin lat&Lon (degree)"; OrinAlt "GPS Orin Altitude (m)"; SamTime "Sample Time (s)"
      mask Help: eval('sharedhelp(''UDP_20100_PX4SilRecv'')');
  UDP_30100_TrueSimRecv : Subsystem  mask{CopterID=1, SamTime=-1}
      mask prompts: SamTime "Sample Time (s)"
      mask Help: eval('sharedhelp(''UDP_30100_TrueSimRecv'')');
  UDP_40100_RflyPx4Recv : Subsystem  mask{CopterID=1, SamTime=-1}
      mask prompts: SamTime "Sample Time (s)"
      mask Help: eval('sharedhelp(''UDP_40100_RflyPx4Recv'')');
  getTerrainAltData : MATLAB Function  TreatAsAtomicUnit=on
      mask help: 根据输入的X和Y坐标获取指定位置的地形高度数据。
  sendUE4CMD : MATLAB Function  TreatAsAtomicUnit=on  mask(RflySendUE4CMD){}
      mask help: 向RflySim3D发送控制台命令
  sendUE4ExtAct : Subsystem
      mask Help: eval('sharedhelp(''sendUE4ExtAct'')');
      mask Display: image('UE_Logo.jpg');
  sendUE4Pos2Ground : Subsystem
      mask Help: eval('sharedhelp(''sendUE4Pos2Ground'')');
      mask Display: image('UE_Logo.jpg');
  sendUE4PosFull : Subsystem
      mask Help: eval('sharedhelp(''sendUE4PosFull'')');
      mask Display: image('UE_Logo.jpg');

== system pixhawk_slib_adv/3DOutput ==
  3DType : Inport
  ActuatorToUE : Inport  Port=2
  6DOF : Inport  Port=3
  Bus Selector : BusSelector  OutputSignals=Ve,Xe,Eular(rad),DCM,wb,AccB,PosGPS
  Clock1 : Clock
  Vehile3DModel : Subsystem
  VehileInfo60d : Outport
  wires:
  Bus Selector/4 -> Vehile3DModel/9(<DCM>)  "<DCM>"
  Bus Selector/5 -> Vehile3DModel/6(<wb>)  "<wb>"
  Bus Selector/2 -> Vehile3DModel/7(<Xe>)  "<Xe>"
  3DType/1 -> Vehile3DModel/1(vehicleType)
  ActuatorToUE/1 -> Vehile3DModel/2(ActuatorToUE)
  Clock1/1 -> Vehile3DModel/3(runnedTime)
  Bus Selector/3 -> Vehile3DModel/4(<AngEuler>)  "<Eular(rad)>"
  Bus Selector/1 -> Vehile3DModel/8(<Ve>)  "<Ve>"
  Bus Selector/6 -> Vehile3DModel/5(<AccB>)  "<AccB>"
  6DOF/1 -> Bus Selector/1
  Bus Selector/7 -> Vehile3DModel/10(PosGps)  "<PosGPS>"
  Vehile3DModel/1(VehileInfo60d) -> VehileInfo60d/1

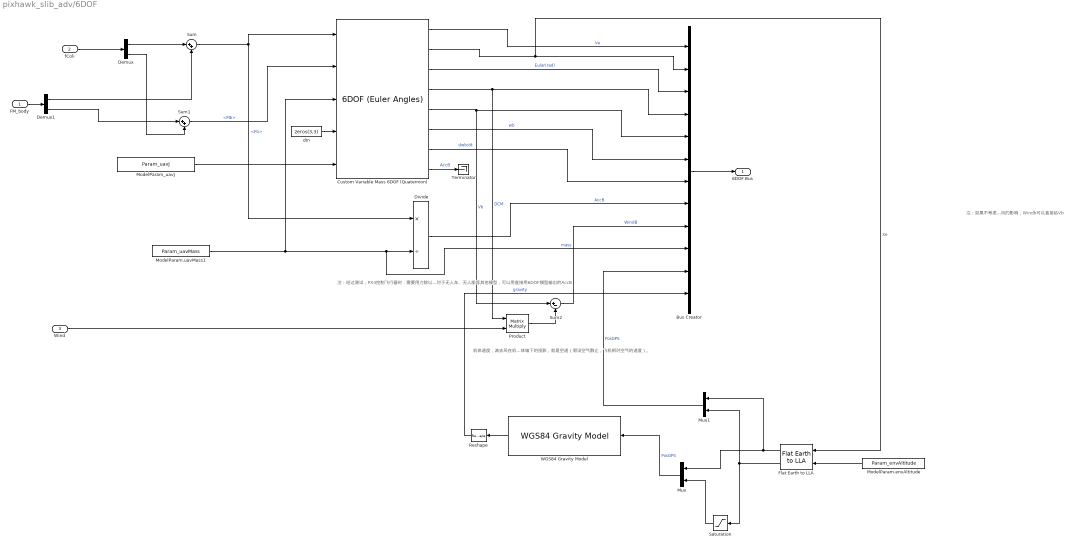
== system pixhawk_slib_adv/6DOF ==
  note: 注：如果不考虑风的影响，Windb可以直接给Vb
  note: 注：经过测试，PX4控制飞行器时，需要用力除以力矩的加速度去生成加速度计的数据，对于无人车、无人船等其他模型，可以用直接用6DOF模型输出的AccB
  note: 机体速度，减去风在机体轴下的投影，就是空速（假设空气静止，飞机相对空气的速度）。
  FM_body : Inport  PortDimensions=6
  fColi : Inport  Port=2  PortDimensions=6
  Wind : Inport  Port=3  PortDimensions=3
  Bus Creator : BusCreator  Inputs=12
  Custom Variable Mass 6DOF (Quaternion) : shared6dof/6DOF (Euler Angles)  units=Metric (MKS)  mtype=Custom Variable  rep=Quaternion  xme_0=Init_PosE  Vm_0=Init_VelB  eul_0=Init_AngEuler  pm_0=Init_RateB  mass_0=ModelParam_uavMass  mass_e=0.5  mass_f=2.0  inertia=ModelParam_uavJ  inertia_e=eye(3)  inertia_f=2*eye(3)  k_quat=1.0  vre_flag=off  abi_flag=off
      settings: SourceProductBaseCode=AE
  Demux : Demux  Outputs=2
  Demux1 : Demux  Outputs=2
  Divide : Product  Inputs=*/
  Flat Earth to LLA : aerolibtransform2/Flat Earth to LLA  units=Metric (MKS)  ptype=Earth (WGS84)  F=1/298.257223563  R=6378137  LL0=Param_GPSLatLong  psi=0
  ModelParam.envAltitude : Constant  Value=Param_envAltitude
  ModelParam.uavMass1 : Constant  Value=Param_uavMass
  ModelParam_uavJ : Constant  Value=Param_uavJ
  Mux : Mux  Inputs=2
  Mux1 : Mux  Inputs=2
  Product : Product  Multiplication=Matrix(*)
  Reshape : Reshape
  Saturation : Saturate  UpperLimit=100000  LowerLimit=0
  Sum : Sum  Inputs=|++
  Sum1 : Sum  Inputs=|++
  Sum2 : Sum  Inputs=|+-
  Terminator : Terminator
  "WGS84 Gravity Model " : aerolibobsolete/WGS84 Gravity Model   model=WGS84 Taylor Series  units=Metric (MKS)  no_atmos=on  precessing=on  jd_loc=off  month=October  day=10  year=2004  no_centrifugal=on  action=Warning
      settings: SourceProductName=Aerospace Blockset  SourceProductBaseCode=AE
  dm : Constant  Value=zeros(3,3)
  6DOF Bus : Outport
  wires:
  Demux1/1 -> Sum/2
  FM_body/1 -> Demux1/1
  Demux/2 -> Sum1/2
  Demux/1 -> Sum/1
  fColi/1 -> Demux/1
  Custom Variable Mass 6DOF (Quaternion)/7 -> Bus Creator/7  "dwb/dt"
  Bus Creator/1 -> 6DOF Bus/1
  Custom Variable Mass 6DOF (Quaternion)/6 -> Bus Creator/6  "wb"
  Sum1/1 -> Custom Variable Mass 6DOF (Quaternion)/2  "<Mb>"
  Sum/1 -> Divide/1, Custom Variable Mass 6DOF (Quaternion)/1  "<Fb>"
  Custom Variable Mass 6DOF (Quaternion)/8 -> Terminator/1  "AccB"
  Custom Variable Mass 6DOF (Quaternion)/4 -> Product/1, Bus Creator/4  "DCM"
  Custom Variable Mass 6DOF (Quaternion)/3 -> Bus Creator/3  "Eular(rad)"
  Custom Variable Mass 6DOF (Quaternion)/1 -> Bus Creator/1  "Ve"
  ModelParam.uavMass1/1 -> Bus Creator/10, Divide/2, Custom Variable Mass 6DOF (Quaternion)/3  "mass"
  Divide/1 -> Bus Creator/8  "AccB"
  Wind/1 -> Product/2
  Product/1 -> Sum2/2
  Sum2/1 -> Bus Creator/9  "WindB"
  dm/1 -> Custom Variable Mass 6DOF (Quaternion)/4
  ModelParam_uavJ/1 -> Custom Variable Mass 6DOF (Quaternion)/5
  Mux1/1 -> Bus Creator/11  "PosGPS"
  Mux/1 -> "WGS84 Gravity Model "/1  "PosGPS"
  ModelParam.envAltitude/1 -> Flat Earth to LLA/2
  Saturation/1 -> Mux/2
  Flat Earth to LLA/2 -> Saturation/1, Mux1/2
  Custom Variable Mass 6DOF (Quaternion)/5 -> Bus Creator/5, Sum2/1  "Vb"
  "WGS84 Gravity Model "/1 -> Reshape/1
  Reshape/1 -> Bus Creator/12  "gravity"
  Flat Earth to LLA/1 -> Mux1/1, Mux/1
  Custom Variable Mass 6DOF (Quaternion)/2 -> Flat Earth to LLA/1, Bus Creator/2  "Xe"
  Demux1/2 -> Sum1/1

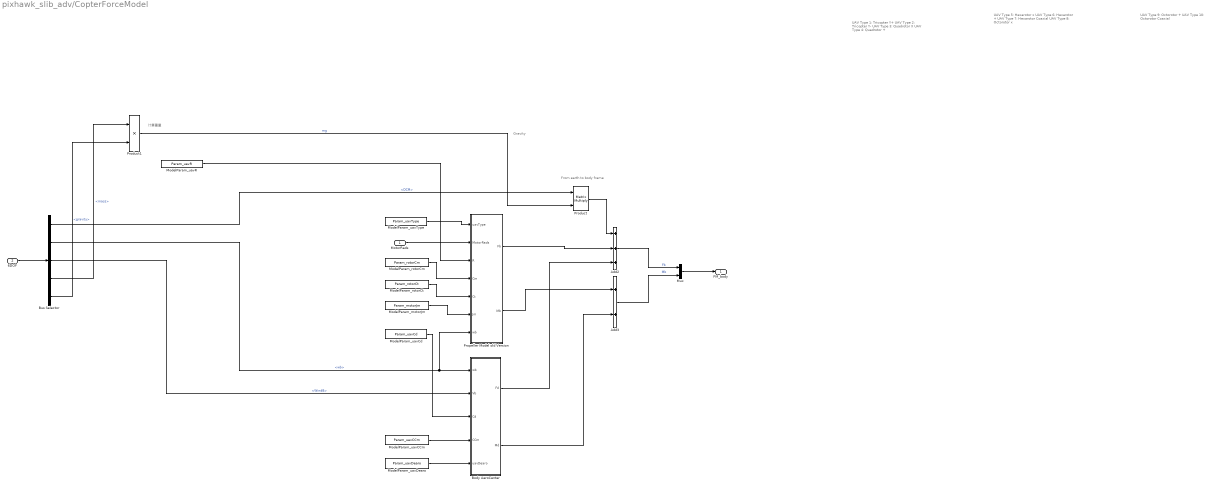
== system pixhawk_slib_adv/CopterForceModel ==
  note: 计算重量
  note: From earth to body frame
  note: Gravity
  note: UAV Type 1: Tricopter Y+
      |
      | UAV Type 2: Tricopter Y-
      |
      | UAV Type 3: Quadrotor X
      |
      | UAV Type 4: Quadrotor +
  note: UAV Type 5: Hexarotor x
      |
      | UAV Type 6: Hexarotor +
      |
      | UAV Type 7: Hexarotor Coaxial
      |
      | UAV Type 8: Octorotor x
  note: UAV Type 9: Octorotor +
      |
      | UAV Type 10: Octorotor Coaxial
  MotorRads : Inport
  6DOF : Inport  Port=2
  Add2 : Sum  Inputs=+++
  Add3 : Sum
  Body AeroCenter : MATLAB Function  TreatAsAtomicUnit=on
  Bus Selector : BusSelector  OutputSignals=DCM,wb,WindB,mass,gravity
  ModelParam_motorJm : Constant  Value=Param_motorJm
  ModelParam_rotorCm : Constant  Value=Param_rotorCm
  ModelParam_rotorCt : Constant  Value=Param_rotorCt
  ModelParam_uavCCm : Constant  Value=Param_uavCCm
  ModelParam_uavCd : Constant  Value=Param_uavCd
  ModelParam_uavDearo : Constant  Value=Param_uavDearo
  ModelParam_uavR : Constant  Value=Param_uavR
  ModelParam_uavType : Constant  Value=Param_uavType
  Mux : Mux  Inputs=2
  Product : Product  Multiplication=Matrix(*)
  Product1 : Product
  Propeller Model old Version : MATLAB Function  TreatAsAtomicUnit=on
  FM_body : Outport
  wires:
  Mux/1 -> FM_body/1
  Bus Selector/5 -> Product1/2  "<gravity>"
  Bus Selector/4 -> Product1/1  "<mass>"
  Product1/1 -> Product/2  "mg"
  Bus Selector/3 -> Body AeroCenter/2(Vb)  "<WindB>"
  ModelParam_rotorCt/1 -> Propeller Model old Version/5(Ct)
  ModelParam_rotorCm/1 -> Propeller Model old Version/4(Cm)
  Propeller Model old Version/1(Fb) -> Add2/2
  Propeller Model old Version/2(Mb) -> Add3/1
  ModelParam_motorJm/1 -> Propeller Model old Version/6(Jm)
  MotorRads/1 -> Propeller Model old Version/2(MotorRads)
  ModelParam_uavType/1 -> Propeller Model old Version/1(uavType)
  ModelParam_uavR/1 -> Propeller Model old Version/3(R)
  ModelParam_uavDearo/1 -> Body AeroCenter/5(uavDearo)
  6DOF/1 -> Bus Selector/1
  ModelParam_uavCCm/1 -> Body AeroCenter/4(CCm)
  Bus Selector/2 -> Propeller Model old Version/7(wb), Body AeroCenter/1(wb)  "<wb>"
  ModelParam_uavCd/1 -> Body AeroCenter/3(Cd)
  Bus Selector/1 -> Product/1  "<DCM>"
  Product/1 -> Add2/1
  Add2/1 -> Mux/1  "Fb"
  Add3/1 -> Mux/2  "Mb"
  Body AeroCenter/1(Fd) -> Add2/3
  Body AeroCenter/2(Md) -> Add3/2

== system pixhawk_slib_adv/CopterGroundModel ==
  note: GroundSupportModel
  note: From Earth to body frame
  note: 计算重量
  "tZ " : Inport
  6DOF : Inport  Port=2
  Bus Selector : BusSelector  OutputSignals=Xe,Ve,Eular(rad),DCM,wb,mass,gravity
  Direction Cosine Matrix to Quaternions : sharedtransform/Direction Cosine Matrix  to Quaternions
      settings: SourceProductName=Aerospace Blockset  SourceProductBaseCode=AE
  Direction Cosine Matrix to Quaternions1 : sharedtransform/Direction Cosine Matrix  to Quaternions
      settings: SourceProductName=Aerospace Blockset  SourceProductBaseCode=AE
  Euler to DCM : aerolibtransform2/Wind Angles to  Direction Cosine Matrix
      settings: SourceProductName=Aerospace Blockset  SourceProductBaseCode=AE
  Ground Model : MATLAB Function  TreatAsAtomicUnit=on
  Mux : Mux  Inputs=2
  OnGroundFaceup : Subsystem
  Product : Product  Multiplication=Matrix(*)
  Product1 : Product
  Quaternion Inverse : aerolibutil/Quaternion Inverse
      settings: SourceProductName=Aerospace Blockset
  Quaternion Multiplication : aerolibutil/Quaternion Multiplication
  FM : Outport
  wires:
  "tZ "/1 -> Ground Model/6(TerrainIn)
  Ground Model/2(M1) -> Mux/2  "Mb"
  Product/1 -> Mux/1  "Fb"
  Quaternion Multiplication/1 -> Ground Model/5(Quet)
  Quaternion Inverse/1 -> Quaternion Multiplication/1
  Direction Cosine Matrix to Quaternions1/1 -> Quaternion Inverse/1
  Euler to DCM/1 -> Direction Cosine Matrix to Quaternions1/1
  Direction Cosine Matrix to Quaternions/1 -> Quaternion Multiplication/2
  Ground Model/1(F1) -> Product/2
  Bus Selector/4 -> Direction Cosine Matrix to Quaternions/1, Product/1  "<DCM>"
  Bus Selector/5 -> Ground Model/2(wb)  "<wb>"
  6DOF/1 -> Bus Selector/1
  Bus Selector/2 -> Ground Model/4(Ve)  "<Ve>"
  Bus Selector/1 -> Ground Model/3(Xe)  "<Xe>"
  Bus Selector/3 -> OnGroundFaceup/1(Eular(rad))  "<Eular(rad)>"
  OnGroundFaceup/1(y) -> Euler to DCM/1
  Product1/1 -> Ground Model/1(mg)  "mg"
  Bus Selector/6 -> Product1/1  "<mass>"
  Bus Selector/7 -> Product1/2  "<gravity>"
  Mux/1 -> FM/1
